simulink model "untitled1"  (R2016b)
settings: Solver=VariableStepAuto  StartTime=0.0  StopTime=10.0  RelTol=1e-3
libraries: fuzblock x1
settings Model: Creator=salee  LastModifiedBy=salee

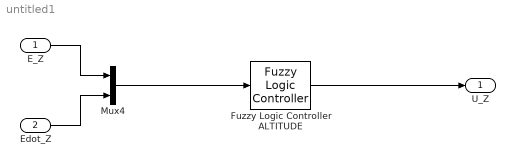
== system untitled1 ==
  E_Z : Inport  OutputFunctionCall=on
  Edot_Z : Inport  Port=2  OutputFunctionCall=on
  "Fuzzy Logic Controller ALTITUDE " : fuzblock/Fuzzy Logic  Controller  fis='Quadrotor.fis'
  Mux4 : Mux  Inputs=2
  U_Z : Outport
  wires:
  E_Z/1 -> Mux4/1
  Edot_Z/1 -> Mux4/2
  Mux4/1 -> "Fuzzy Logic Controller ALTITUDE "/1
  "Fuzzy Logic Controller ALTITUDE "/1 -> U_Z/1
